simulink model "watertank"  (Simulink 8.5)
settings: Solver=ode45  StartTime=0.0  StopTime=1000  RelTol=1e-3
settings Model: Creator=stefano  LastModifiedBy=stefano
settings DataIOCC: SignalLoggingSaveFormat=Dataset
settings OptimizationCC: ExpressionDepthLimit=128
settings DebuggingCC: UnderspecifiedInitializationDetection=Simplified  MergeDetectMultiDrivingBlocksExec=error  FcnCallInpInsideContextMsg=EnableAllAsError  StateNameClashWarn=none
settings GRTTargetCC: CombineOutputUpdateFcns=on  GRTInterface=off

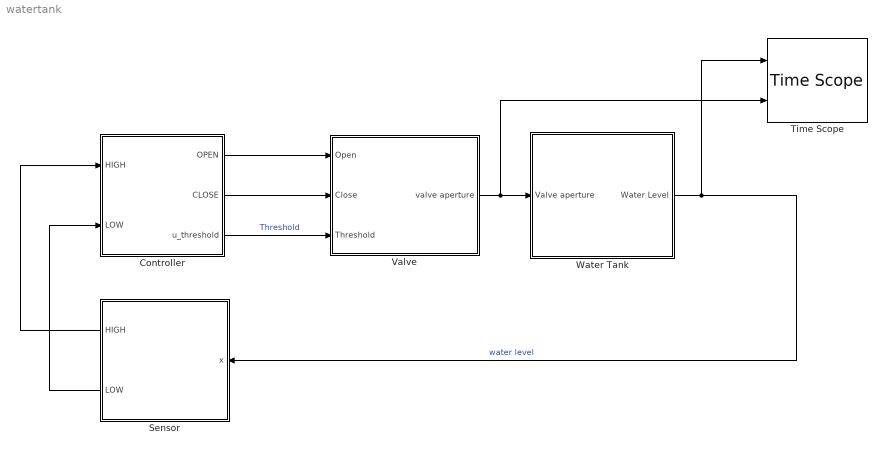
== system watertank ==
  "Controller " : Stateflow chart  TreatAsAtomicUnit=on
  Sensor : Stateflow chart  TreatAsAtomicUnit=on
  Time Scope : TimeScope  DefaultConfigurationName=spbscopes.TimeScopeBlockCfg  NumInputPorts=2
  Valve : Subsystem
  Water Tank : Subsystem
  wires:
  "Controller "/3(u_threshold) -> Valve/3(Threshold)  "Threshold"
  Sensor/1(HIGH) -> "Controller "/1(HIGH)
  Sensor/2(LOW) -> "Controller "/2(LOW)
  "Controller "/1(OPEN) -> Valve/1(Open)
  "Controller "/2(CLOSE) -> Valve/2(Close)
  Water Tank/1(Water Level) -> Time Scope/1, Sensor/1(x)  "water level"
  Valve/1(valve aperture) -> Time Scope/2, Water Tank/1(Valve aperture)

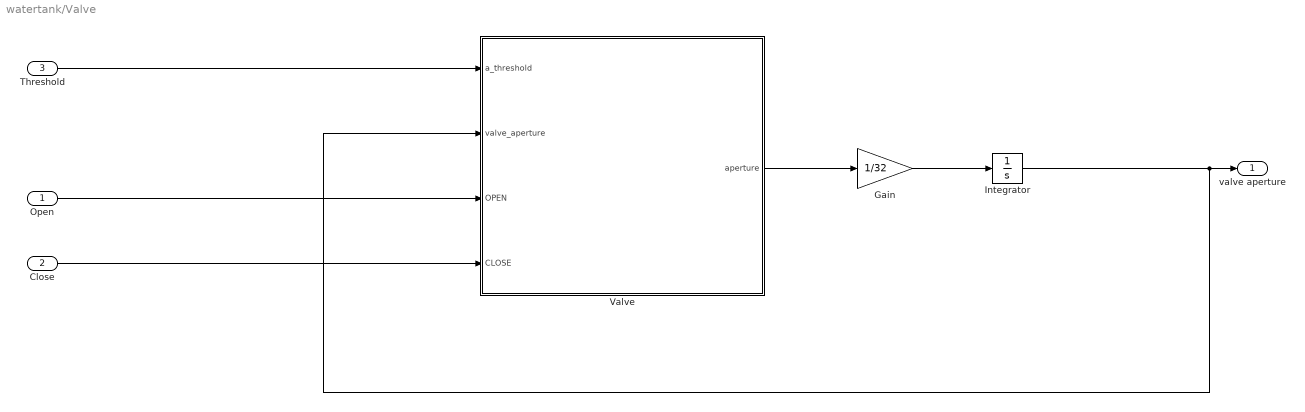
== system watertank/Valve ==
  Open : Inport
  Close : Inport  Port=2
  Threshold : Inport  Port=3
  Gain : Gain  Gain=1/32
  Integrator : Integrator  LimitOutput=on
  "Valve " : Stateflow chart  TreatAsAtomicUnit=on
  valve aperture : Outport
  wires:
  Threshold/1 -> "Valve "/1(a_threshold)
  "Valve "/1(aperture) -> Gain/1
  Gain/1 -> Integrator/1
  Integrator/1 -> valve aperture/1, "Valve "/2(valve_aperture)
  Open/1 -> "Valve "/3(OPEN)
  Close/1 -> "Valve "/4(CLOSE)

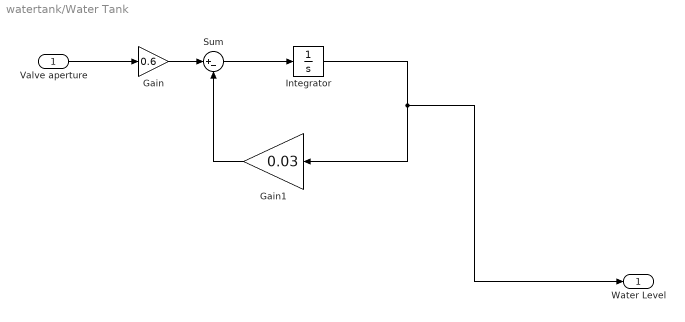
== system watertank/Water Tank ==
  Valve aperture : Inport
  Gain : Gain  Gain=0.6
  Gain1 : Gain  Gain=0.03
  Integrator : Integrator
  Sum : Sum  Inputs=|+-
  Water Level : Outport
  wires:
  Integrator/1 -> Water Level/1, Gain1/1
  Sum/1 -> Integrator/1
  Valve aperture/1 -> Gain/1
  Gain1/1 -> Sum/2
  Gain/1 -> Sum/1

== stateflow chart Valve/Valve  ==
  settings: updateMethod=DISCRETE  sampleTime=0.1
  state OPENING
    entry: aperture = 1
  state IDLE
    entry:  aperture = 0;
  state CLOSING
    entry: aperture = -1
  OPENING -> CLOSING [order 2] : [CLOSE == 1]
  IDLE -> OPENING [order 2] : [OPEN == 1]
  OPENING -> IDLE [order 1] : [valve_aperture>=a_threshold]
  CLOSING -> OPENING [order 2] : [OPEN == 1]
  (default) -> IDLE
  CLOSING -> IDLE [order 1] : [valve_aperture<=0]
  IDLE -> CLOSING [order 1] : [CLOSE==1]
  data: a_threshold input single; aperture output double; valve_aperture input double; OPEN input boolean; CLOSE input boolean

== stateflow chart Sensor ==
  settings: updateMethod=DISCRETE  sampleTime=0.1
  state EMPTY
    entry: LOW= false;
    entry: HIGH = false;
    entry: t=0;
    during: t= t+1;
  state FULL
    entry: HIGH= false;
    entry: LOW = false;
    entry: t=0;
    during: t= t+1;
  state SAFE
    entry: HIGH = false;
    entry: LOW = false;
  state EMPTY1
    entry: LOW = true;
  state FULL1
    entry: HIGH= true;
    ;
  EMPTY1 -> EMPTY
  EMPTY -> EMPTY1 [order 2] : [x<=Low & t >=5 ]
  FULL1 -> FULL
  FULL -> FULL1 [order 3] : [x>=High & t >=5]
  FULL -> EMPTY [order 2] : [x<=Low]
  SAFE -> EMPTY [order 2] : [x<=Low]
  EMPTY -> SAFE [order 1] : [x>Low]
  SAFE -> FULL [order 1] : [x>= High]
  FULL -> SAFE [order 1] : [x<= High]
  (default) -> SAFE
  data: Low constant single =5.5; x input double; High constant single =8; t local double; HIGH output boolean; LOW output boolean

== stateflow chart Controller  ==
  settings: updateMethod=DISCRETE  sampleTime=0.1
  state INCREASE
    entry: u_threshold = u_threshold + (u_threshold * 0.1)
    entry:OPEN = true;
    entry: CLOSE = false;
  state DECREASE
    entry: u_threshold = u_threshold - (u_threshold * 0.3);
    entry: CLOSE = true;
    entry: OPEN = false;
  state ACTIVE
    entry: u_threshold = 0.7
  state NOTHING
    entry: OPEN = false;
    entry: CLOSE = false;
  (default) -> ACTIVE
  ACTIVE -> INCREASE : [ LOW==true ]
  NOTHING -> INCREASE [order 1] : [ LOW == true]
  INCREASE -> NOTHING
  DECREASE -> NOTHING
  NOTHING -> DECREASE [order 2] : [ HIGH == true]
  data: OPEN output boolean; CLOSE output boolean; Low constant double =5.5; High constant double =8; u_threshold output double; HIGH input boolean; LOW input boolean
